simulink model "velo_id_gain"  (R2025b)
settings: Solver=VariableStepAuto  StartTime=0.0  StopTime=10.0  RelTol=1e-3
model workspace (MAT data in the model file):
  u_ini = Simulink.Parameter
  u_ini.Complexity = 'real'
  u_ini.Dimensions = [0 0]
  u_ini.DataType = 'auto'
  u_ref = Simulink.Parameter
  u_ref.Complexity = 'real'
  u_ref.Dimensions = [0 0]
  u_ref.DataType = 'auto'
libraries: arduino_io_lib x4
settings Model: Creator=nttha  LastModifiedBy=trong

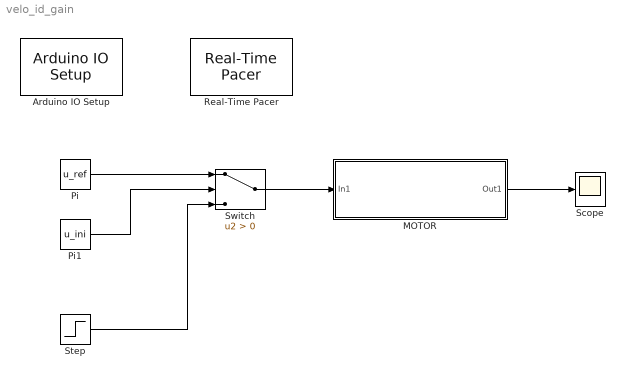
== system velo_id_gain ==
  Arduino IO Setup : arduino_io_lib/Arduino IO Setup  Priority=3  arduinoVar=Temporary arduino variable: Arduino1  workspaceVarName=a  comPort=COM3
      settings: SourceProductName=Arduino IO Library
  MOTOR : Subsystem
  Pi : Constant  Value=u_ref  OutDataTypeStr=Inherit: Inherit via back propagation
  Pi1 : Constant  Value=u_ini  OutDataTypeStr=Inherit: Inherit via back propagation
  Real-Time Pacer : arduino_io_lib/Real-Time Pacer  simTimePerRealTime=1
      settings: SourceProductName=Arduino IO Library
  Scope : Scope
      settings: ActiveDisplayYMinimum=-1.4999999999999996  ActiveDisplayYMaximum=13.5
  Step : Step  SampleTime=0
  Switch : Switch  Criteria=u2 > Threshold  SaturateOnIntegerOverflow=off  InputSameDT=off
  wires:
  Pi/1 -> Switch/1
  Pi1/1 -> Switch/2
  Step/1 -> Switch/3
  Switch/1 -> MOTOR/1(In1)
  MOTOR/1(Out1) -> Scope/1

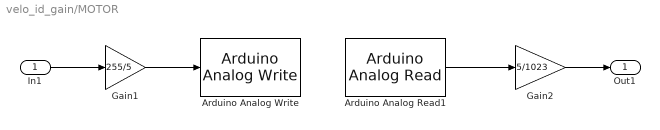
== system velo_id_gain/MOTOR ==
  In1 : Inport
  Arduino Analog Read1 : arduino_io_lib/Arduino Analog Read  arduinoVar=Temporary arduino variable: Arduino1  arduinoPin=0  T=0.02
      settings: SourceProductName=Arduino IO Library
  Arduino Analog Write : arduino_io_lib/Arduino Analog Write  arduinoVar=Temporary arduino variable: Arduino1  arduinoPin=3  T=0.02
      settings: SourceProductName=Arduino IO Library
  Gain1 : Gain  Gain=255/5
  Gain2 : Gain  Gain=5/1023
  Out1 : Outport
  wires:
  In1/1 -> Gain1/1
  Arduino Analog Read1/1 -> Gain2/1
  Gain1/1 -> Arduino Analog Write/1
  Gain2/1 -> Out1/1
